simulink model "ex3_linear_nonlinear_control"  (R2024b)
settings: Solver=FixedStepAuto  StartTime=0.0  StopTime=Tf  FixedStep=dt  RelTol=1e-3
undefined symbols (not defined in the file or in its folder): q0
libraries: robotmobilelib x4
settings Model: Creator=fiore  LastModifiedBy=fiore

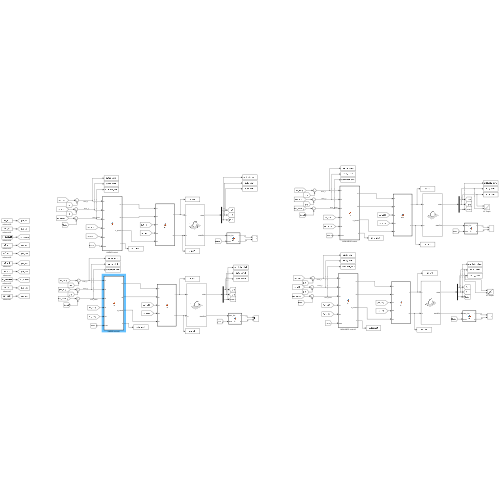
[thumbnail: Simulink's stored preview of the top-level diagram]
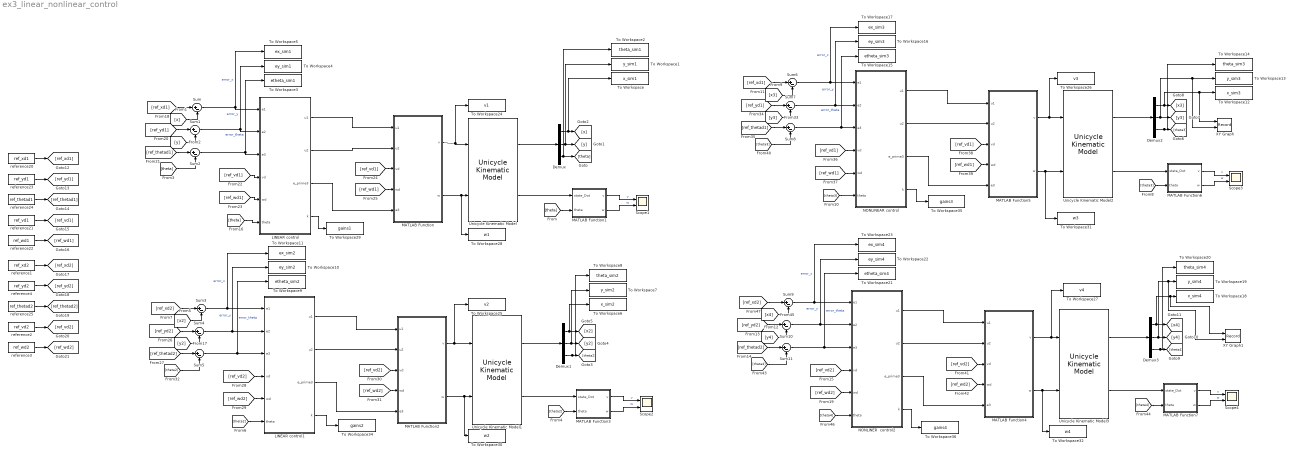
== system ex3_linear_nonlinear_control ==
  Demux{,1..3} (4 alike) : Demux  Outputs=3
  LINEAR control : MATLAB Function  TreatAsAtomicUnit=on
  LINEAR control1 : MATLAB Function  TreatAsAtomicUnit=on
  MATLAB Function : MATLAB Function  TreatAsAtomicUnit=on
  MATLAB Function1 : MATLAB Function  TreatAsAtomicUnit=on
  MATLAB Function2 : MATLAB Function  TreatAsAtomicUnit=on
  MATLAB Function3 : MATLAB Function  TreatAsAtomicUnit=on
  MATLAB Function4 : MATLAB Function  TreatAsAtomicUnit=on
  MATLAB Function5 : MATLAB Function  TreatAsAtomicUnit=on
  MATLAB Function6 : MATLAB Function  TreatAsAtomicUnit=on
  MATLAB Function7 : MATLAB Function  TreatAsAtomicUnit=on
  NONLINEAR control : MATLAB Function  TreatAsAtomicUnit=on
  NONLINER  control2 : MATLAB Function  TreatAsAtomicUnit=on
  Scope{1..4} (4 alike) : Scope  NumInputPorts=2
  Sum{,1..11} (12 alike) : Sum  Inputs=|+-
  To Workspace : ToWorkspace  VariableName=x_sim1  SaveFormat=Timeseries  SampleTime=-1
  To Workspace1 : ToWorkspace  VariableName=y_sim1  SaveFormat=Timeseries  SampleTime=-1
  To Workspace10 : ToWorkspace  VariableName=ey_sim2  SaveFormat=Timeseries  SampleTime=-1
  To Workspace11 : ToWorkspace  VariableName=ex_sim2  SaveFormat=Timeseries  SampleTime=-1
  To Workspace12 : ToWorkspace  VariableName=x_sim3  SaveFormat=Timeseries  SampleTime=-1
  To Workspace13 : ToWorkspace  VariableName=y_sim3  SaveFormat=Timeseries  SampleTime=-1
  To Workspace14 : ToWorkspace  VariableName=theta_sim3  SaveFormat=Timeseries  SampleTime=-1
  To Workspace15 : ToWorkspace  VariableName=etheta_sim3  SaveFormat=Timeseries  SampleTime=-1
  To Workspace16 : ToWorkspace  VariableName=ey_sim3  SaveFormat=Timeseries  SampleTime=-1
  To Workspace17 : ToWorkspace  VariableName=ex_sim3  SaveFormat=Timeseries  SampleTime=-1
  To Workspace18 : ToWorkspace  VariableName=x_sim4  SaveFormat=Timeseries  SampleTime=-1
  To Workspace19 : ToWorkspace  VariableName=y_sim4  SaveFormat=Timeseries  SampleTime=-1
  To Workspace2 : ToWorkspace  VariableName=theta_sim1  SaveFormat=Timeseries  SampleTime=-1
  To Workspace20 : ToWorkspace  VariableName=theta_sim4  SaveFormat=Timeseries  SampleTime=-1
  To Workspace21 : ToWorkspace  VariableName=etheta_sim4  SaveFormat=Timeseries  SampleTime=-1
  To Workspace22 : ToWorkspace  VariableName=ey_sim4  SaveFormat=Timeseries  SampleTime=-1
  To Workspace23 : ToWorkspace  VariableName=ex_sim4  SaveFormat=Timeseries  SampleTime=-1
  To Workspace24 : ToWorkspace  VariableName=v1  SaveFormat=Timeseries  SampleTime=-1
  To Workspace25 : ToWorkspace  VariableName=v2  SaveFormat=Timeseries  SampleTime=-1
  To Workspace26 : ToWorkspace  VariableName=v3  SaveFormat=Timeseries  SampleTime=-1
  To Workspace27 : ToWorkspace  VariableName=v4  SaveFormat=Timeseries  SampleTime=-1
  To Workspace28 : ToWorkspace  VariableName=w1  SaveFormat=Timeseries  SampleTime=-1
  To Workspace29 : ToWorkspace  VariableName=gains1  SaveFormat=Timeseries  SampleTime=-1
  To Workspace3 : ToWorkspace  VariableName=etheta_sim1  SaveFormat=Timeseries  SampleTime=-1
  To Workspace30 : ToWorkspace  VariableName=w2  SaveFormat=Timeseries  SampleTime=-1
  To Workspace31 : ToWorkspace  VariableName=w3  SaveFormat=Timeseries  SampleTime=-1
  To Workspace32 : ToWorkspace  VariableName=w4  SaveFormat=Timeseries  SampleTime=-1
  To Workspace34 : ToWorkspace  VariableName=gains2  SaveFormat=Timeseries  SampleTime=-1
  To Workspace35 : ToWorkspace  VariableName=gains3  SaveFormat=Timeseries  SampleTime=-1
  To Workspace36 : ToWorkspace  VariableName=gains4  SaveFormat=Timeseries  SampleTime=-1
  To Workspace4 : ToWorkspace  VariableName=ey_sim1  SaveFormat=Timeseries  SampleTime=-1
  To Workspace5 : ToWorkspace  VariableName=ex_sim1  SaveFormat=Timeseries  SampleTime=-1
  To Workspace6 : ToWorkspace  VariableName=x_sim2  SaveFormat=Timeseries  SampleTime=-1
  To Workspace7 : ToWorkspace  VariableName=y_sim2  SaveFormat=Timeseries  SampleTime=-1
  To Workspace8 : ToWorkspace  VariableName=theta_sim2  SaveFormat=Timeseries  SampleTime=-1
  To Workspace9 : ToWorkspace  VariableName=etheta_sim2  SaveFormat=Timeseries  SampleTime=-1
  Unicycle Kinematic Model : robotmobilelib/Unicycle Kinematic Model  VehicleInputs=Vehicle Speed & Heading Angular Velocity  WheelRadius=0.05  WheelSpeedRange=[-Inf Inf]  InitialState=q0(1,:)  SimulateUsing=Interpreted execution
  Unicycle Kinematic Model1 : robotmobilelib/Unicycle Kinematic Model  VehicleInputs=Vehicle Speed & Heading Angular Velocity  WheelRadius=0.05  WheelSpeedRange=[-Inf Inf]  InitialState=q0(2,:)  SimulateUsing=Interpreted execution
  Unicycle Kinematic Model2 : robotmobilelib/Unicycle Kinematic Model  VehicleInputs=Vehicle Speed & Heading Angular Velocity  WheelRadius=0.05  WheelSpeedRange=[-Inf Inf]  InitialState=q0(1,:)  SimulateUsing=Interpreted execution
  Unicycle Kinematic Model3 : robotmobilelib/Unicycle Kinematic Model  VehicleInputs=Vehicle Speed & Heading Angular Velocity  WheelRadius=0.05  WheelSpeedRange=[-Inf Inf]  InitialState=q0(2,:)  SimulateUsing=Interpreted execution
  XY Graph : Record  FileSettingsInternal="{\"entries\":[{\"content\":{\"excelSettings\":{\"content\":{},\"type\":\"Streamout.ExcelSettings\"}},\"type\":\"Streamout.FileSettingStorage\",\"uuid\":\"\"}],\"packageUris\":[\"http:\\/\\/schema.mathworks.com\\/mf0\\/streamout_blocks\\/R2020a\"],\"version\":\"1.0\"}"  Layout=[1 1]  SignalsInternal="{\"entries\":[{\"content\":{\"signals\":[{\"content\":{\"blockPath\":[],\"dimensions\":[1],\"domain\":\"\",\"lineColor\":\"#a2142f\",\"plots\":[ 1 ],\"port\":1,\"sid\":[\"\"],\"signalID\":1,\"signalName\":\"Demux2:1\"},\"type\":\"RecordBlkView.Signal\",\"uuid\":\"\"},{\"content\":{\"blockPath\":[],\"dimensions\":[1],\"domain\":\"\",\"lineColor\":\"#139fff\",\"plots\":[ 1 ],\"port\":2,\"sid\":[\"\"],\"signalID\":2,\"signalName\":\"Demux2:2\"},\"type\":\"RecordBlkView.Signal\",\"uuid\":\"\"}]},\"type\":\"RecordBlkView.InputSignals\",\"uuid\":\"\"}],\"packageUris\":[\"http:\\/\\/schema.mathworks.com\\/mf0\\/streamout_blocks\\/R2020a\"],\"version\":\"1.0\"}"  VisualizationBindings="{\"xyplotplugin\":{\"info\":[{\"series\":[{\"bindingParametersList\":[{\"parameter\":\"X-Axis\",\"signalID\":1,\"signalName\":\"Demux2:1\"},{\"parameter\":\"Y-Axis\",\"signalID\":2,\"signalName\":\"Demux2:2\"}],\"seriesID\":0}],\"subplotID\":1}]}}"  CompatibilityTag=XY
  XY Graph1 : Record  FileSettingsInternal="{\"entries\":[{\"content\":{\"excelSettings\":{\"content\":{},\"type\":\"Streamout.ExcelSettings\"}},\"type\":\"Streamout.FileSettingStorage\",\"uuid\":\"\"}],\"packageUris\":[\"http:\\/\\/schema.mathworks.com\\/mf0\\/streamout_blocks\\/R2020a\"],\"version\":\"1.0\"}"  Layout=[1 1]  SignalsInternal="{\"entries\":[{\"content\":{\"signals\":[{\"content\":{\"blockPath\":[],\"dimensions\":[1],\"domain\":\"\",\"lineColor\":\"#a2142f\",\"plots\":[ 1 ],\"port\":1,\"sid\":[\"\"],\"signalID\":1,\"signalName\":\"Demux3:1\"},\"type\":\"RecordBlkView.Signal\",\"uuid\":\"\"},{\"content\":{\"blockPath\":[],\"dimensions\":[1],\"domain\":\"\",\"lineColor\":\"#139fff\",\"plots\":[ 1 ],\"port\":2,\"sid\":[\"\"],\"signalID\":2,\"signalName\":\"Demux3:2\"},\"type\":\"RecordBlkView.Signal\",\"uuid\":\"\"}]},\"type\":\"RecordBlkView.InputSignals\",\"uuid\":\"\"}],\"packageUris\":[\"http:\\/\\/schema.mathworks.com\\/mf0\\/streamout_blocks\\/R2020a\"],\"version\":\"1.0\"}"  VisualizationBindings="{\"xyplotplugin\":{\"info\":[{\"series\":[{\"bindingParametersList\":[{\"parameter\":\"X-Axis\",\"signalID\":1,\"signalName\":\"Demux3:1\"},{\"parameter\":\"Y-Axis\",\"signalID\":2,\"signalName\":\"Demux3:2\"}],\"seriesID\":0}],\"subplotID\":1}]}}"  CompatibilityTag=XY
  reference1 : FromWorkspace  VariableName=ref_xd2
  reference2 : FromWorkspace  VariableName=ref_vd2
  reference20 : FromWorkspace  VariableName=ref_xd1
  reference21 : FromWorkspace  VariableName=ref_vd1
  reference22 : FromWorkspace  VariableName=ref_wd1
  reference23 : FromWorkspace  VariableName=ref_yd1
  reference24 : FromWorkspace  VariableName=ref_thetad1
  reference25 : FromWorkspace  VariableName=ref_thetad2
  reference3 : FromWorkspace  VariableName=ref_wd2
  reference4 : FromWorkspace  VariableName=ref_yd2
  wires:
  Unicycle Kinematic Model/1 -> Demux/1
  [ref_xd1] -> Sum/1
  Sum/1 -> LINEAR control/1(e1), To Workspace5/1  "error_x"
  MATLAB Function1/1(v) -> Scope1/1  "v"
  [theta] -> MATLAB Function1/2(theta)
  MATLAB Function1/2(w) -> Scope1/2  "w"
  Unicycle Kinematic Model/2 -> MATLAB Function1/1(state_Dot)
  Demux/3 -> [theta], To Workspace2/1
  Demux/1 -> [x], To Workspace/1
  Demux/2 -> [y], To Workspace1/1
  [ref_vd1] -> LINEAR control/4(vd)
  Sum1/1 -> To Workspace4/1, LINEAR control/2(e2)  "error_y"
  [ref_yd1] -> Sum1/1
  [ref_thetad1] -> Sum2/1
  Sum2/1 -> To Workspace3/1, LINEAR control/3(e3)  "error_theta"
  [x] -> Sum/2
  [y] -> Sum1/2
  [theta] -> Sum2/2
  MATLAB Function/1(v) -> To Workspace24/1, Unicycle Kinematic Model/1
  MATLAB Function/2(w) -> To Workspace28/1, Unicycle Kinematic Model/2
  LINEAR control/1(u1) -> MATLAB Function/1(u1)
  LINEAR control/2(u2) -> MATLAB Function/2(u2)
  LINEAR control/3(e_prime3) -> MATLAB Function/5(e3)
  reference20/1 -> [ref_xd1]
  reference23/1 -> [ref_yd1]
  reference24/1 -> [ref_thetad1]
  reference21/1 -> [ref_vd1]
  reference22/1 -> [ref_wd1]
  [theta] -> LINEAR control/6(theta)
  [ref_wd1] -> LINEAR control/5(wd)
  [ref_vd1] -> MATLAB Function/3(vd)
  [ref_wd1] -> MATLAB Function/4(wd)
  reference25/1 -> [ref_thetad2]
  reference2/1 -> [ref_vd2]
  reference4/1 -> [ref_yd2]
  reference3/1 -> [ref_wd2]
  reference1/1 -> [ref_xd2]
  [theta2] -> LINEAR control1/6(theta)
  LINEAR control1/3(e_prime3) -> MATLAB Function2/5(e3)
  LINEAR control1/1(u1) -> MATLAB Function2/1(u1)
  MATLAB Function2/2(w) -> To Workspace30/1, Unicycle Kinematic Model1/2
  LINEAR control1/2(u2) -> MATLAB Function2/2(u2)
  [ref_xd2] -> Sum3/1
  [ref_thetad2] -> Sum5/1
  [ref_vd2] -> MATLAB Function2/3(vd)
  [ref_wd2] -> LINEAR control1/5(wd)
  [ref_wd2] -> MATLAB Function2/4(wd)
  Sum5/1 -> To Workspace9/1, LINEAR control1/3(e3)  "error_theta"
  Demux1/2 -> To Workspace7/1, [y2]
  [x2] -> Sum3/2
  Sum4/1 -> To Workspace10/1, LINEAR control1/2(e2)  "error_y"
  [ref_yd2] -> Sum4/1
  [theta2] -> Sum5/2
  Demux1/3 -> To Workspace8/1, [theta2]
  Demux1/1 -> To Workspace6/1, [x2]
  [ref_vd2] -> LINEAR control1/4(vd)
  [theta2] -> MATLAB Function3/2(theta)
  Unicycle Kinematic Model1/1 -> Demux1/1
  Unicycle Kinematic Model1/2 -> MATLAB Function3/1(state_Dot)
  Sum3/1 -> To Workspace11/1, LINEAR control1/1(e1)  "error_x"
  MATLAB Function2/1(v) -> To Workspace25/1, Unicycle Kinematic Model1/1
  [y2] -> Sum4/2
  MATLAB Function3/2(w) -> Scope2/2  "w"
  MATLAB Function3/1(v) -> Scope2/1  "v"
  [theta3] -> NONLINEAR control/6(theta)
  NONLINEAR control/3(e_prime3) -> MATLAB Function5/5(e3)
  NONLINEAR control/1(u1) -> MATLAB Function5/1(u1)
  MATLAB Function5/2(w) -> To Workspace31/1, Unicycle Kinematic Model2/2
  NONLINEAR control/2(u2) -> MATLAB Function5/2(u2)
  [ref_xd1] -> Sum6/1
  [ref_thetad1] -> Sum8/1
  [ref_vd1] -> MATLAB Function5/3(vd)
  [ref_wd1] -> NONLINEAR control/5(wd)
  [ref_wd1] -> MATLAB Function5/4(wd)
  Sum8/1 -> To Workspace15/1, NONLINEAR control/3(e3)  "error_theta"
  Demux2/2 -> [y3], XY Graph/2, To Workspace13/1
  [x3] -> Sum6/2
  Sum7/1 -> To Workspace16/1, NONLINEAR control/2(e2)  "error_y"
  [ref_yd1] -> Sum7/1
  [theta3] -> Sum8/2
  Demux2/3 -> To Workspace14/1, [theta3]
  Demux2/1 -> XY Graph/1, To Workspace12/1, [x3]
  [ref_vd1] -> NONLINEAR control/4(vd)
  MATLAB Function6/2(w) -> Scope3/2  "w"
  MATLAB Function6/1(v) -> Scope3/1  "v"
  [theta3] -> MATLAB Function6/2(theta)
  Unicycle Kinematic Model2/1 -> Demux2/1
  Unicycle Kinematic Model2/2 -> MATLAB Function6/1(state_Dot)
  Sum6/1 -> To Workspace17/1, NONLINEAR control/1(e1)  "error_x"
  MATLAB Function5/1(v) -> To Workspace26/1, Unicycle Kinematic Model2/1
  [y3] -> Sum7/2
  Sum9/1 -> To Workspace23/1, NONLINER  control2/1(e1)  "error_x"
  Unicycle Kinematic Model3/2 -> MATLAB Function7/1(state_Dot)
  [theta4] -> MATLAB Function7/2(theta)
  Unicycle Kinematic Model3/1 -> Demux3/1
  [y4] -> Sum10/2
  [ref_vd2] -> NONLINER  control2/4(vd)
  Demux3/3 -> To Workspace20/1, [theta4]
  [ref_yd2] -> Sum10/1
  [x4] -> Sum9/2
  [theta4] -> Sum11/2
  MATLAB Function4/1(v) -> To Workspace27/1, Unicycle Kinematic Model3/1
  Sum11/1 -> To Workspace21/1, NONLINER  control2/3(e3)  "error_theta"
  [ref_vd2] -> MATLAB Function4/3(vd)
  NONLINER  control2/2(u2) -> MATLAB Function4/2(u2)
  [ref_thetad2] -> Sum11/1
  Sum10/1 -> To Workspace22/1, NONLINER  control2/2(e2)  "error_y"
  NONLINER  control2/1(u1) -> MATLAB Function4/1(u1)
  NONLINER  control2/3(e_prime3) -> MATLAB Function4/5(e3)
  [ref_wd2] -> MATLAB Function4/4(wd)
  [ref_xd2] -> Sum9/1
  MATLAB Function4/2(w) -> To Workspace32/1, Unicycle Kinematic Model3/2
  [ref_wd2] -> NONLINER  control2/5(wd)
  [theta4] -> NONLINER  control2/6(theta)
  MATLAB Function7/2(w) -> Scope4/2  "w"
  MATLAB Function7/1(v) -> Scope4/1  "v"
  Demux3/2 -> XY Graph1/2, To Workspace19/1, [y4]
  Demux3/1 -> XY Graph1/1, To Workspace18/1, [x4]
  LINEAR control/4(k) -> To Workspace29/1
  NONLINEAR control/4(k) -> To Workspace35/1
  LINEAR control1/4(k) -> To Workspace34/1
  NONLINER  control2/4(k) -> To Workspace36/1

== matlab function ex3_linear_nonlinear_control/MATLAB Function4 ==
  data: u1 input; v output; u2 input; vd input; wd input; w output; e3 input
function [v, w] = fcn(u1, u2, vd, wd, e3)
v = vd*cos(e3) - u1;
w = wd - u2;
end

== matlab function ex3_linear_nonlinear_control/MATLAB Function ==
  data: u1 input; v output; u2 input; vd input; wd input; w output; e3 input
function [v, w] = fcn(u1, u2, vd, wd, e3)
v = vd*cos(e3) - u1;
w = wd - u2;
end

== matlab function ex3_linear_nonlinear_control/MATLAB Function3 ==
  data: state_Dot input; v output; w output; theta input
function [v,w] = fcn(state_Dot,theta)

w = state_Dot(3);
v = state_Dot(1)/cos(theta);

end

== matlab function ex3_linear_nonlinear_control/MATLAB Function6 ==
  data: state_Dot input; v output; w output; theta input
function [v,w] = fcn(state_Dot,theta)

w = state_Dot(3);
v = state_Dot(1)/cos(theta);

end

== matlab function ex3_linear_nonlinear_control/MATLAB Function7 ==
  data: state_Dot input; v output; w output; theta input
function [v,w] = fcn(state_Dot,theta)

w = state_Dot(3);
v = state_Dot(1)/cos(theta);

end

== matlab function ex3_linear_nonlinear_control/LINEAR control1 ==
  data: e1 input; e2 input; e3 input; u1 output; vd input; wd input; u2 output; theta input; e_prime3 output; k output
function [u1, u2, e_prime3, k] = fcn(e1, e2, e3, vd, wd, theta)

a = 70;
xi = 0.7;
k1 = 2*xi*a;
k3 = k1;
k2 = (a^2 - wd)/vd;
k = [k1, k2, k3];

e = [e1, e2, e3]';
T = [cos(theta), sin(theta), 0;
    -sin(theta), cos(theta), 0;
    0, 0, 1];
e_prime = T*e;
e_prime3 = e_prime(3);

u1 = - k1*e_prime(1);
u2 = - k2*e_prime(2) - k3*e_prime(3);
end

== matlab function ex3_linear_nonlinear_control/LINEAR control ==
  data: e1 input; e2 input; e3 input; u1 output; vd input; wd input; u2 output; theta input; e_prime3 output; k output
function [u1, u2, e_prime3, k] = fcn(e1, e2, e3, vd, wd, theta)

a = 70;
xi = 0.7;
k1 = 2*xi*a;
k3 = k1;
k2 = (a^2 - wd)/vd;
k = [k1, k2, k3];

e = [e1, e2, e3]';
T = [cos(theta), sin(theta), 0;
    -sin(theta), cos(theta), 0;
    0, 0, 1];
e_prime = T*e;
e_prime3 = e_prime(3);

u1 = - k1*e_prime(1);
u2 = - k2*e_prime(2) - k3*e_prime(3);
end

== matlab function ex3_linear_nonlinear_control/MATLAB Function2 ==
  data: u1 input; v output; u2 input; vd input; wd input; w output; e3 input
function [v, w] = fcn(u1, u2, vd, wd, e3)
v = vd*cos(e3) - u1;
w = wd - u2;
end

== matlab function ex3_linear_nonlinear_control/MATLAB Function1 ==
  data: state_Dot input; v output; w output; theta input
function [v,w] = fcn(state_Dot,theta)

w = state_Dot(3);
v = state_Dot(1)/cos(theta);

end

== matlab function ex3_linear_nonlinear_control/NONLINEAR control ==
  data: e1 input; e2 input; e3 input; u1 output; vd input; wd input; u2 output; theta input; e_prime3 output; k output
function [u1, u2, e_prime3, k] = fcn(e1, e2, e3, vd, wd, theta)
a = 10;
k1 = (a^2 - wd)/vd;
k3 = k1;
k2 = 50;
k = [k1, k2, k3];

e = [e1, e2, e3]';
T = [cos(theta), sin(theta), 0;
    -sin(theta), cos(theta), 0;
    0, 0, 1];
e_prime = T*e;
e_prime3 = e_prime(3);

u1 = - k1*e_prime(1);
u2 = - k2*vd*(sinc(e_prime3))*e_prime(2) - k3*e_prime3;
end

== matlab function ex3_linear_nonlinear_control/MATLAB Function5 ==
  data: u1 input; v output; u2 input; vd input; wd input; w output; e3 input
function [v, w] = fcn(u1, u2, vd, wd, e3)
v = vd*cos(e3) - u1;
w = wd - u2;
end

== matlab function ex3_linear_nonlinear_control/NONLINER  control2 ==
  data: e1 input; e2 input; e3 input; u1 output; vd input; wd input; u2 output; theta input; e_prime3 output; k output
function [u1, u2, e_prime3, k] = fcn(e1, e2, e3, vd, wd, theta)
a = 27;
k1 = (a^2 - wd)/vd;
k3 = k1;
k2 = 200;
k = [k1, k2, k3];

e = [e1, e2, e3]';
T = [cos(theta), sin(theta), 0;
    -sin(theta), cos(theta), 0;
    0, 0, 1];
e_prime = T*e;
e_prime3 = e_prime(3);

u1 = - k1*e_prime(1);
u2 = - k2*vd*(sinc(e_prime3))*e_prime(2) - k3*e_prime3;
end
